simulink model "P1s2"  (R2015b)
settings: Solver=FixedStepAuto  StartTime=0.0  StopTime=5  RelTol=1e-3
libraries: powerlib x10
settings Model: Creator=xmax1946  LastModifiedBy=xmax1946

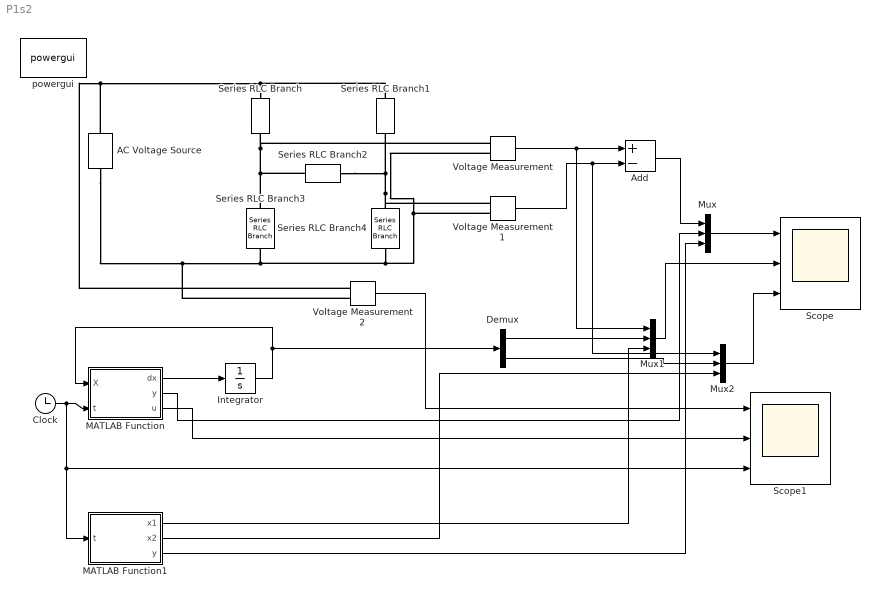
== system P1s2 ==
  AC Voltage Source : powerlib/Electrical Sources/AC Voltage Source  Amplitude=10  Phase=0  Frequency=.159154  SampleTime=0  Measurements=None  BusType=swing  Pref=10e3  Qref=0  Qmin=-inf  Qmax=+inf
  Add : Sum  Inputs=+-
  Clock : Clock
  Demux : Demux  Outputs=2
  Integrator : Integrator  InitialCondition=[10;5]
  MATLAB Function : MATLAB Function  TreatAsAtomicUnit=on
  MATLAB Function1 : MATLAB Function  TreatAsAtomicUnit=on
  Mux : Mux  Inputs=3
  Mux1 : Mux  Inputs=3
  Mux2 : Mux  Inputs=3
  Scope : Scope  NumInputPorts=3
  Scope1 : Scope  NumInputPorts=3
  Series RLC Branch : powerlib/Elements/Series RLC Branch  LConnTagsString=__new0  RConnTagsString=__new0  BranchType=R  Resistance=5  Inductance=1e-3  SetiL0=off  InitialCurrent=0  Capacitance=1e-6  Setx0=off  InitialVoltage=0  Measurements=None
  Series RLC Branch1 : powerlib/Elements/Series RLC Branch  LConnTagsString=__new0  RConnTagsString=__new0  BranchType=R  Resistance=10  Inductance=1e-3  SetiL0=off  InitialCurrent=0  Capacitance=1e-6  Setx0=off  InitialVoltage=0  Measurements=None
  Series RLC Branch2 : powerlib/Elements/Series RLC Branch  LConnTagsString=__new0  RConnTagsString=__new0  BranchType=R  Resistance=1  Inductance=1e-3  SetiL0=off  InitialCurrent=0  Capacitance=1e-6  Setx0=off  InitialVoltage=0  Measurements=None
  Series RLC Branch3 : powerlib/Elements/Series RLC Branch  LConnTagsString=__new0  RConnTagsString=__new0  BranchType=C  Resistance=1  Inductance=1e-3  SetiL0=off  InitialCurrent=0  Capacitance=1  Setx0=on  InitialVoltage=10  Measurements=None
  Series RLC Branch4 : powerlib/Elements/Series RLC Branch  LConnTagsString=__new0  RConnTagsString=__new0  BranchType=C  Resistance=1  Inductance=1e-3  SetiL0=off  InitialCurrent=0  Capacitance=2  Setx0=on  InitialVoltage=5  Measurements=None
  Voltage Measurement : powerlib/Measurements/Voltage Measurement  PhasorSimulation=off  OutputType=Complex  PSBequivalent=0
  Voltage Measurement1 : powerlib/Measurements/Voltage Measurement  PhasorSimulation=off  OutputType=Complex  PSBequivalent=0
  Voltage Measurement2 : powerlib/Measurements/Voltage Measurement  PhasorSimulation=off  OutputType=Complex  PSBequivalent=0
  powergui : powerlib/powergui  Priority=1  SimulationMode=Discrete  SolverType=Tustin/Backward Euler (TBE)  SampleTime=50e-6  frequency=60  SPID=off  DisableSnubberDevices=off  DisableRonSwitches=off  DisableVfSwitches=off  SwTol=0  DisplayEquations=off  Interpol=off  ExternalGateDelay=off  methode=off  Ts=10  FunctionMessages=off  echomessages=off  HookPort=off  EnableUseOfTLC=off  x0status=blocks  frequencyindice=0.159154  Pbase=100e6  ErrMax=1e-4  Iterations=50  UnitsV=kV  UnitsW=MW  buscounter=0  RestoreLinks=warning  ResistiveCurrentMeasurement=off  Frange=[0:2:500]  Ylog=off  Xlog=on  ShowGrid=off  save=off  variable=ZData  structure=0  ZoomFFT=off  StartTime=0.0  cycles=1  DisplayStyle=1  fundamental=60  FreqAxis=off  MaxFrequency=1000  frequencyindicesteady=1  RmsSteady=1  display=off
  wires:
  Voltage Measurement/1 -> Mux1/1, Add/1
  Voltage Measurement1/1 -> Mux2/1, Add/2
  MATLAB Function/1(dx) -> Integrator/1
  Integrator/1 -> Demux/1, MATLAB Function/1(X)
  Clock/1 -> Scope1/3, MATLAB Function1/1(t), MATLAB Function/2(t)
  Mux/1 -> Scope/1
  Demux/1 -> Mux1/2
  Mux1/1 -> Scope/2
  Demux/2 -> Mux2/2
  Mux2/1 -> Scope/3
  MATLAB Function1/1(x1) -> Mux1/3
  MATLAB Function1/2(x2) -> Mux2/3
  MATLAB Function1/3(y) -> Mux/3
  Voltage Measurement2/1 -> Scope1/1
  MATLAB Function/3(u) -> Scope1/2
  Add/1 -> Mux/1
  MATLAB Function/2(y) -> Mux/2
  connections:
  Series RLC Branch3/LConn1 -- Series RLC Branch2/RConn1 -- Voltage Measurement/LConn1 -- Series RLC Branch/RConn1
  Series RLC Branch4/LConn1 -- Series RLC Branch2/LConn1 -- Series RLC Branch1/RConn1 -- Voltage Measurement1/LConn1
  Series RLC Branch1/LConn1 -- Voltage Measurement2/LConn1 -- AC Voltage Source/RConn1 -- Series RLC Branch/LConn1
  Series RLC Branch4/RConn1 -- Voltage Measurement1/LConn2 -- Voltage Measurement/LConn2 -- Voltage Measurement2/LConn2 -- AC Voltage Source/LConn1 -- Series RLC Branch3/RConn1

== matlab function P1s2/MATLAB Function1 ==
  data: x1 output; x2 output; t input; y output
function [x1,x2,y] = f2(t)
x1=(440*sin(t))/769 - (6400*cos(t))/5383 + 10*exp(-(7*t)/8)*(cosh((969^(1/2)*t)/40) - (13*969^(1/2)*sinh((969^(1/2)*t)/40))/969) + (6400*exp(-(7*t)/8)*(cosh((969^(1/2)*t)/40) + (21*969^(1/2)*sinh((969^(1/2)*t)/40))/1292))/5383 + (200*969^(1/2)*exp(-(7*t)/8)*sinh((969^(1/2)*t)/40))/969;
x2= 5*exp(-(7*t)/8)*(cosh((969^(1/2)*t)/40) + (13*969^(1/2)*sinh((969^(1/2)*t)/40))/969) - (670*sin(t))/5383 - (4600*cos(t))/5383 + (4600*exp(-(7*t)/8)*(cosh((969^(1/2)*t)/40) + (313*969^(1/2)*sinh((969^(1/2)*t)/40))/7429))/5383 + (200*969^(1/2)*exp(-(7*t)/8)*sinh((969^(1/2)*t)/40))/969;
y=(3750*sin(t))/5383 - (1800*cos(t))/5383 + 10*exp(-(7*t)/8)*(cosh((969^(1/2)*t)/40) - (13*969^(1/2)*sinh((969^(1/2)*t)/40))/969) - 5*exp(-(7*t)/8)*(cosh((969^(1/2)*t)/40) + (13*969^(1/2)*sinh((969^(1/2)*t)/40))/969) + (6400*exp(-(7*t)/8)*(cosh((969^(1/2)*t)/40) + (21*969^(1/2)*sinh((969^(1/2)*t)/40))/1292))/5383 - (4600*exp(-(7*t)/8)*(cosh((969^(1/2)*t)/40) + (313*969^(1/2)*sinh((969^(1/2)*t)/40))/7429))/5383;

== matlab function P1s2/MATLAB Function ==
  data: dx output; X input; y output; t input; u output
function [dx,y,u] = f(X,t)
R1=5;
R2=10;
R3=1;
C1=1;
C2=2;

A=[(-1/C1)*((R3+R1)/(R3*R1)),1/(R3*C1);1/(C2*R3),(-1/C2)*((R2+R3)/(R2*R3))];
B=[1/(R1*C1);1/(R2*C2)];
C=[1,-1];
u=10*sin(t);
dx=A*X+B*u;
y=C*X;
